simulink model "ChargingInterfaceCtrl"  (R2024a)
settings: Solver=VariableStepAuto  StartTime=0.0  StopTime=10.0  RelTol=1e-3
settings Model: DataDictionary=BMS_System_Arch_dict.sldd  Creator=ghourabi  LastModifiedBy=ghourabi

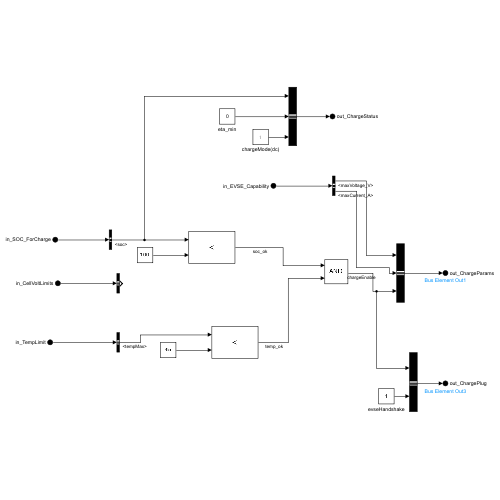
[thumbnail: Simulink's stored preview of the top-level diagram]
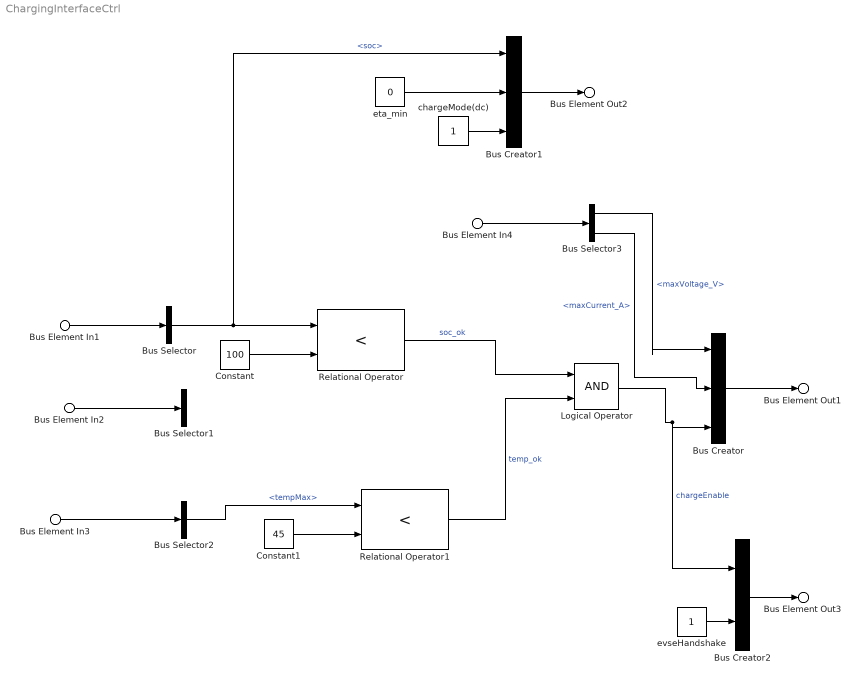
== system ChargingInterfaceCtrl ==
  Bus Element In1 : Inport  PortName=in_SOC_ForCharge
  Bus Element In2 : Inport  Port=2  PortName=in_CellVoltLimits
  Bus Element In3 : Inport  Port=3  PortName=in_TempLimit
  Bus Element In4 : Inport  Port=4  PortName=in_EVSE_Capability
  Bus Creator : BusCreator  Inputs=3
  Bus Creator1 : BusCreator  Inputs=3
  Bus Creator2 : BusCreator  Inputs=2
  Bus Selector : BusSelector  OutputSignals=soc
  Bus Selector1 : BusSelector  OutputSignals=maxCellVoltage
  Bus Selector2 : BusSelector  OutputSignals=tempMax
  Bus Selector3 : BusSelector  OutputSignals=maxVoltage_V,maxCurrent_A
  Constant : Constant  Value=100
  Constant1 : Constant  Value=45
  Logical Operator : Logic  AllPortsSameDT=off  OutDataTypeStr=boolean
  Relational Operator : RelationalOperator  Operator=<  OutDataTypeStr=boolean  RndMeth=Simplest  InputSameDT=off
  Relational Operator1 : RelationalOperator  Operator=<  OutDataTypeStr=boolean  RndMeth=Simplest  InputSameDT=off
  chargeMode(dc) : Constant
  eta_min : Constant  Value=0
  evseHandshake : Constant
  Bus Element Out1 : Outport  PortName=out_ChargeParams
  Bus Element Out2 : Outport  Port=2  PortName=out_ChargeStatus
  Bus Element Out3 : Outport  Port=3  PortName=out_ChargePlug
  wires:
  Bus Element In1/1 -> Bus Selector/1
  Bus Element In2/1 -> Bus Selector1/1
  Bus Element In4/1 -> Bus Selector3/1
  Bus Element In3/1 -> Bus Selector2/1
  Bus Selector/1 -> Bus Creator1/1, Relational Operator/1  "<soc>"
  Constant/1 -> Relational Operator/2
  Relational Operator/1 -> Logical Operator/1  "soc_ok"
  Relational Operator1/1 -> Logical Operator/2  "temp_ok"
  Constant1/1 -> Relational Operator1/2
  Bus Selector2/1 -> Relational Operator1/1  "<tempMax>"
  Logical Operator/1 -> Bus Creator2/1, Bus Creator/3  "chargeEnable"
  Bus Selector3/1 -> Bus Creator/1  "<maxVoltage_V>"
  Bus Selector3/2 -> Bus Creator/2  "<maxCurrent_A>"
  Bus Creator/1 -> Bus Element Out1/1
  eta_min/1 -> Bus Creator1/2
  chargeMode(dc)/1 -> Bus Creator1/3
  Bus Creator1/1 -> Bus Element Out2/1
  evseHandshake/1 -> Bus Creator2/2
  Bus Creator2/1 -> Bus Element Out3/1
